simulink model "current_example"  (Simulink 7.6)
settings: Solver=ode45  StartTime=0.0  StopTime=10.0  RelTol=1e-3
libraries: QB_pacer_lib x1, qbmove_library x1
settings Model: Creator=felipe  LastModifiedBy=felipe

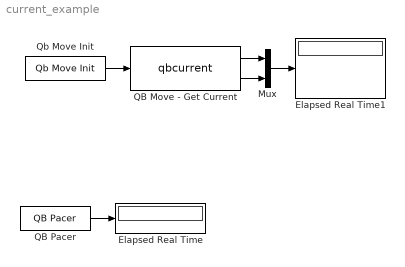
== system current_example ==
  Elapsed Real Time : Display
      settings: Decimation=2
  Elapsed Real Time1 : Display
      settings: Decimation=2
  Mux : Mux  Inputs=2
  QB Move - Get Current : S-Function  AncestorBlock=qbmove_library/qbmove  FunctionName=qbcurrent  Parameters=ID, DAISY_CHAINING  EnableBusSupport=off  mask(qb move){ID=65, CONTROL_MODE=Prime Movers Positions, DAISY_CHAINING=off}
      mask prompts: CONTROL_MODE "Input Type"; DAISY_CHAINING "Daisy Chaining Enable"
      mask help:
      | This block allows you to obtain the currents from the QB Move.
      | It needs an handle from QB Move Init block.
      mask StyleString: edit,popup(Prime Movers Positions|Equilibrium Position and Stiffness Preset),checkbox
      mask TabNameString: Options,Options,Options
  QB Pacer : QB_pacer_lib/QB Pacer  simTimePerRealTime=1
  Qb Move Init : qbmove_library/Qb Move Init  NUMBER_OF_COM='/dev/tty.usbserial-DAWQ5P42'
  wires:
  QB Pacer/1 -> Elapsed Real Time/1
  Qb Move Init/1 -> QB Move - Get Current/1
  Mux/1 -> Elapsed Real Time1/1
  QB Move - Get Current/1 -> Mux/1
  QB Move - Get Current/2 -> Mux/2
